simulink model "Mpc_SimMechanics_with_standing"  (R2017b)
settings: Solver=ode45  StartTime=0  StopTime=10  FixedStep=0.0005  EnableMultiTasking=on
InitFcn:
  | isSim = 1;
  | 
  | PreFunctions.CustomInitFcn_with_standing;
  | PreFunctions.simulationInitFcn_with_standing;
undefined symbols (not defined in the file): alpha_x, alpha_y, DiagnosticCodes, DynamicMatrixLibrary, motorPositions, motorVelocities, pelvisPosition, pelvisVelocity, sample_time, X, Y, Z
libraries: sm_lib x170, nesl_utility x75, Contact_Forces_Lib x6, ComponentLibrary x5, xpcrtudplib x2, slrtlib x1
(part 8 of 8)

== system Mpc_SimMechanics_with_standing/Cassie/Cassie Simulation/Cassie Right Leg/Hip Roll Drive ==
  Bus Element In : Inport  PortName=InBus  Element=torque
  Actual Torque Scaling : Gain  Gain=-gearRatio
  Constant1 : Constant  Value=0
  Constant2 : Constant  Value=0  OutDataTypeStr=uint16
  Constant3 : Constant  Value=0
  Constant4 : Constant  Value=peakTorque*gearRatio
  Constant5 : Constant  Value=gearRatio
  Gear Constraint : sm_lib/Gears and Couplings/Gears/Common Gear Constraint  GearType=External  SpecificationType=CenterDistanceRatio  CenterDistance=1e-6  CenterDistanceUnits=m  GearRatio=gearRatio  BaseGearRadius=10.0  BaseGearRadiusUnits=cm  FollGearRadius=10.0  FollGearRadiusUnits=cm  AssemblyGearRotation=Free
      settings: SourceProductName=Simscape Multibody  SourceProductBaseCode=MS
  Gear Constraint Offset : sm_lib/Frames and Transforms/Rigid Transform  TranslationMethod=StandardAxis  TranslationStandardOffset=1e-6  TranslationLengthUnit=m  TranslationStandardAxis=+Y  TranslationCartesianOffset=[0 0 0]  TranslationROffset=0  TranslationROffsetUnits=m  TranslationZOffset=0  TranslationZOffsetUnits=m  TranslationThetaOffset=0  TranslationThetaOffsetUnits=deg  RotationMethod=None  RotationAngleUnits=deg  RotationStandardAxis=+Z  RotationAngle=0.0  RotationArbitraryAxis=[0 0 1]  FollAlignAxisA=+X  BaseAlignAxisA=+Y  FollAlignAxisB=+Y  BaseAlignAxisB=+Z  RotationSequenceAxes=FollowerAxes  RotationSequence=XYX  RotationSequenceAngles=[0 0 0]  RotationSequenceAnglesUnits=deg  RotationMatrix=[1 0 0; 0 1 0; 0 0 1]
  Input Revolute Joint : sm_lib/Joints/Revolute Joint  SenseConstraintForce=off  SenseConstraintForceX=off  SenseConstraintForceY=off  SenseConstraintForceZ=off  SenseConstraintTorque=off  SenseConstraintTorqueX=off  SenseConstraintTorqueY=off  SenseConstraintTorqueZ=off  SenseTotalForce=off  SenseTotalForceX=off  SenseTotalForceY=off  SenseTotalForceZ=off  SenseTotalTorque=off  SenseTotalTorqueX=off  SenseTotalTorqueY=off  SenseTotalTorqueZ=off  CompositeWrenchDir=FollowerOnBase  CompositeWrenchFrame=BaseFrame  EquilibriumPosition=0  EquilibriumPositionUnits=rad  SpringStiffness=0  SpringStiffnessUnits=N*m/rad  DampingCoefficient=0  DampingCoefficientUnits=N*m/(rad/s)  TorqueActuationMode=InputTorque  MotionActuationMode=ComputedMotion  SensePosition=off  SenseVelocity=on  SenseAcceleration=off  SenseTorqueForce=off  PositionTargetSpecify=off  PositionTargetPriority=High  PositionTargetValue=0  PositionTargetValueUnits=deg  VelocityTargetSpecify=off  VelocityTargetPriority=High  VelocityTargetValue=0  VelocityTargetValueUnits=rad/s
  MATLAB Function : MATLAB Function  TreatAsAtomicUnit=on
  Output Revolute Joint : sm_lib/Joints/Revolute Joint  SenseConstraintForce=off  SenseConstraintForceX=off  SenseConstraintForceY=off  SenseConstraintForceZ=off  SenseConstraintTorque=off  SenseConstraintTorqueX=off  SenseConstraintTorqueY=off  SenseConstraintTorqueZ=off  SenseTotalForce=off  SenseTotalForceX=off  SenseTotalForceY=off  SenseTotalForceZ=off  SenseTotalTorque=off  SenseTotalTorqueX=off  SenseTotalTorqueY=off  SenseTotalTorqueZ=off  CompositeWrenchDir=FollowerOnBase  CompositeWrenchFrame=BaseFrame  EquilibriumPosition=0  EquilibriumPositionUnits=rad  SpringStiffness=0  SpringStiffnessUnits=N*m/rad  DampingCoefficient=1  DampingCoefficientUnits=N*m/(rad/s)  TorqueActuationMode=NoTorque  MotionActuationMode=ComputedMotion  SensePosition=on  SenseVelocity=on  SenseAcceleration=off  SenseTorqueForce=off  PositionTargetSpecify=on  PositionTargetPriority=High  PositionTargetValue=initialPosition  PositionTargetValueUnits=rad  VelocityTargetSpecify=on  VelocityTargetPriority=High  VelocityTargetValue=initialVelocity  VelocityTargetValueUnits=rad/s
  PS-Simulink Converter : nesl_utility/PS-Simulink Converter  PhysicalDomain=network_engine_domain  SubClassName=ps_output  LeftPortType=input  RightPortType=output  PseudoPeriodic=off  Frequencies=[]  Unit=rad  AffineConversion=off
  PS-Simulink Converter1 : nesl_utility/PS-Simulink Converter  PhysicalDomain=network_engine_domain  SubClassName=ps_output  LeftPortType=input  RightPortType=output  PseudoPeriodic=off  Frequencies=[]  Unit=rad/s  AffineConversion=off
  PS-Simulink Converter2 : nesl_utility/PS-Simulink Converter  PhysicalDomain=network_engine_domain  SubClassName=ps_output  LeftPortType=input  RightPortType=output  PseudoPeriodic=off  Frequencies=[]  Unit=rad/s  AffineConversion=off
  Quantizer : Quantizer  QuantizationInterval=(2*pi)/(encoderResolution*gearRatio)
  Rate Transition : RateTransition  Deterministic=off  InitialCondition=initialPosition  OutPortSampleTimeOpt=Inherit
  Rate Transition1 : RateTransition  Deterministic=off  InitialCondition=initialPosition  OutPortSampleTimeOpt=Inherit
  Rotor Solid : sm_lib/Body Elements/Solid  InertiaType=Custom  Mass=0  MassUnits=kg  CenterOfMass=[0; 0; 0]  CenterOfMassUnits=m  MomentsOfInertia=[0; 0; rotorInertia]  MomentsOfInertiaUnits=kg*m^2  ProductsOfInertia=[0; 0; 0]  ProductsOfInertiaUnits=kg*m^2  DensityBased=on  Density=1000  DensityUnits=kg/m^3  DoExposeReferenceFrame=on  SerializedFrames=<Frames/>  GraphicType=None  MarkerShape=Sphere  MarkerSize=10  GraphicVisPropType=SimpleVisualProperties  GraphicDiffuseColor=[0.5 0.5 0.5]  GraphicSpecularColor=[0.5 0.5 0.5 1.0]  GraphicAmbientColor=[0.15 0.15 0.15 1.0]  GraphicEmissiveColor=[0.0 0.0 0.0 1.0]  GraphicShininess=75  GraphicOpacity=1.0  GeometryShape=Cylinder  RectangleSize=[1 1]  RectangleSizeUnits=m  BrickDimensions=[1 1 1]  BrickDimensionUnits=m  CylinderRadius=1  CylinderRadiusUnits=m  CylinderLength=1  CylinderLengthUnits=m  SphereRadius=1  SphereRadiusUnits=m  EllipsoidRadii=[1 1 1]  EllipsoidRadiiUnits=m  ExtrusionCrossSection=[1 1; -1 1; -1 -1; 1 -1]  ExtrusionCrossSectionUnits=m  ExtrusionLength=1  ExtrusionLengthUnits=m  PolygonNumSides=3  PolygonOuterRadius=1  PolygonOuterRadiusUnits=m  ExtGeomFileType=STEP  ExtGeomFileUnits=m  RevolutionCrossSection=[1 1; 1 -1; 2 -1; 2 1]  RevolutionCrossSectionUnits=m  RevolutionExtent=Full  RevolutionAngle=180  RevolutionAngleUnits=deg
  Simulink-PS Converter : nesl_utility/Simulink-PS Converter  PhysicalDomain=network_engine_domain  SubClassName=ps_input  LeftPortType=input  RightPortType=output  PseudoPeriodic=off  Frequencies=[]  NoiseDistribution=none  NoiseParameters=[]  Unit=N*m  AffineConversion=off  FilteringAndDerivatives=zero  SimscapeFilterOrder=1  InputFilterTimeConstant=0.001  UdotUserProvided=1
  Target Torque Scaling : Gain  Gain=-1/gearRatio
  Base : PMIOPort  Port=1  Side=Left
  Follower : PMIOPort  Port=2  Side=Right
  Bus Element Out3 : Outport  PortName=OutBus  Element=statusWord
  Bus Element Out : Outport  PortName=OutBus  Element=position
  Bus Element Out4 : Outport  PortName=OutBus  Element=velocity
  Bus Element Out2 : Outport  PortName=OutBus  Element=torque
  Bus Element Out1 : Outport  PortName=OutBus  Element=driveTemperature
  Bus Element Out5 : Outport  PortName=OutBus  Element=dcLinkVoltage
  Bus Element Out6 : Outport  PortName=OutBus  Element=torqueLimit
  Bus Element Out7 : Outport  PortName=OutBus  Element=gearRatio
  Pos : Outport  Port=2
  vel : Outport  Port=3
  wires:
  PS-Simulink Converter2/1 -> vel/1, Rate Transition1/1
  Rate Transition1/1 -> Bus Element Out4/1
  Constant5/1 -> Bus Element Out7/1
  Actual Torque Scaling/1 -> Bus Element Out2/1
  Constant4/1 -> Bus Element Out6/1
  Constant3/1 -> Bus Element Out5/1
  Constant1/1 -> Bus Element Out1/1
  Constant2/1 -> Bus Element Out3/1
  Target Torque Scaling/1 -> MATLAB Function/2("torque ")
  PS-Simulink Converter1/1 -> MATLAB Function/1(speed)
  MATLAB Function/1(torque) -> Simulink-PS Converter/1, Actual Torque Scaling/1
  Bus Element In/1 -> Target Torque Scaling/1
  Quantizer/1 -> Bus Element Out/1
  PS-Simulink Converter/1 -> Pos/1, Rate Transition/1
  Rate Transition/1 -> Quantizer/1
  connections:
  Output Revolute Joint/RConn3 -- PS-Simulink Converter2/LConn1
  Input Revolute Joint/LConn1 -- Base/RConn1 -- Gear Constraint Offset/LConn1
  Simulink-PS Converter/RConn1 -- Input Revolute Joint/LConn2
  PS-Simulink Converter1/LConn1 -- Input Revolute Joint/RConn2
  Rotor Solid/RConn1 -- Gear Constraint/LConn1 -- Input Revolute Joint/RConn1
  Output Revolute Joint/RConn1 -- Follower/RConn1 -- Gear Constraint/RConn1
  Output Revolute Joint/LConn1 -- Gear Constraint Offset/RConn1
  Output Revolute Joint/RConn2 -- PS-Simulink Converter/LConn1

== system Mpc_SimMechanics_with_standing/Cassie/Cassie Simulation/Cassie Right Leg/Hip Yaw Drive ==
  Bus Element In : Inport  PortName=InBus  Element=torque
  Actual Torque Scaling : Gain  Gain=-gearRatio
  Constant1 : Constant  Value=0
  Constant2 : Constant  Value=0  OutDataTypeStr=uint16
  Constant3 : Constant  Value=0
  Constant4 : Constant  Value=peakTorque*gearRatio
  Constant5 : Constant  Value=gearRatio
  Gear Constraint : sm_lib/Gears and Couplings/Gears/Common Gear Constraint  GearType=External  SpecificationType=CenterDistanceRatio  CenterDistance=1e-6  CenterDistanceUnits=m  GearRatio=gearRatio  BaseGearRadius=10.0  BaseGearRadiusUnits=cm  FollGearRadius=10.0  FollGearRadiusUnits=cm  AssemblyGearRotation=Free
      settings: SourceProductName=Simscape Multibody  SourceProductBaseCode=MS
  Gear Constraint Offset : sm_lib/Frames and Transforms/Rigid Transform  TranslationMethod=StandardAxis  TranslationStandardOffset=1e-6  TranslationLengthUnit=m  TranslationStandardAxis=+Y  TranslationCartesianOffset=[0 0 0]  TranslationROffset=0  TranslationROffsetUnits=m  TranslationZOffset=0  TranslationZOffsetUnits=m  TranslationThetaOffset=0  TranslationThetaOffsetUnits=deg  RotationMethod=None  RotationAngleUnits=deg  RotationStandardAxis=+Z  RotationAngle=0.0  RotationArbitraryAxis=[0 0 1]  FollAlignAxisA=+X  BaseAlignAxisA=+Y  FollAlignAxisB=+Y  BaseAlignAxisB=+Z  RotationSequenceAxes=FollowerAxes  RotationSequence=XYX  RotationSequenceAngles=[0 0 0]  RotationSequenceAnglesUnits=deg  RotationMatrix=[1 0 0; 0 1 0; 0 0 1]
  Input Revolute Joint : sm_lib/Joints/Revolute Joint  SenseConstraintForce=off  SenseConstraintForceX=off  SenseConstraintForceY=off  SenseConstraintForceZ=off  SenseConstraintTorque=off  SenseConstraintTorqueX=off  SenseConstraintTorqueY=off  SenseConstraintTorqueZ=off  SenseTotalForce=off  SenseTotalForceX=off  SenseTotalForceY=off  SenseTotalForceZ=off  SenseTotalTorque=off  SenseTotalTorqueX=off  SenseTotalTorqueY=off  SenseTotalTorqueZ=off  CompositeWrenchDir=FollowerOnBase  CompositeWrenchFrame=BaseFrame  EquilibriumPosition=0  EquilibriumPositionUnits=rad  SpringStiffness=0  SpringStiffnessUnits=N*m/rad  DampingCoefficient=0  DampingCoefficientUnits=N*m/(rad/s)  TorqueActuationMode=InputTorque  MotionActuationMode=ComputedMotion  SensePosition=off  SenseVelocity=on  SenseAcceleration=off  SenseTorqueForce=off  PositionTargetSpecify=off  PositionTargetPriority=High  PositionTargetValue=0  PositionTargetValueUnits=deg  VelocityTargetSpecify=off  VelocityTargetPriority=High  VelocityTargetValue=0  VelocityTargetValueUnits=rad/s
  MATLAB Function : MATLAB Function  TreatAsAtomicUnit=on
  Output Revolute Joint : sm_lib/Joints/Revolute Joint  SenseConstraintForce=off  SenseConstraintForceX=off  SenseConstraintForceY=off  SenseConstraintForceZ=off  SenseConstraintTorque=off  SenseConstraintTorqueX=off  SenseConstraintTorqueY=off  SenseConstraintTorqueZ=off  SenseTotalForce=off  SenseTotalForceX=off  SenseTotalForceY=off  SenseTotalForceZ=off  SenseTotalTorque=off  SenseTotalTorqueX=off  SenseTotalTorqueY=off  SenseTotalTorqueZ=off  CompositeWrenchDir=FollowerOnBase  CompositeWrenchFrame=BaseFrame  EquilibriumPosition=0  EquilibriumPositionUnits=rad  SpringStiffness=0  SpringStiffnessUnits=N*m/rad  DampingCoefficient=1  DampingCoefficientUnits=N*m/(rad/s)  TorqueActuationMode=NoTorque  MotionActuationMode=ComputedMotion  SensePosition=on  SenseVelocity=on  SenseAcceleration=off  SenseTorqueForce=off  PositionTargetSpecify=on  PositionTargetPriority=High  PositionTargetValue=initialPosition  PositionTargetValueUnits=rad  VelocityTargetSpecify=on  VelocityTargetPriority=High  VelocityTargetValue=initialVelocity  VelocityTargetValueUnits=rad/s
  PS-Simulink Converter : nesl_utility/PS-Simulink Converter  PhysicalDomain=network_engine_domain  SubClassName=ps_output  LeftPortType=input  RightPortType=output  PseudoPeriodic=off  Frequencies=[]  Unit=rad  AffineConversion=off
  PS-Simulink Converter1 : nesl_utility/PS-Simulink Converter  PhysicalDomain=network_engine_domain  SubClassName=ps_output  LeftPortType=input  RightPortType=output  PseudoPeriodic=off  Frequencies=[]  Unit=rad/s  AffineConversion=off
  PS-Simulink Converter2 : nesl_utility/PS-Simulink Converter  PhysicalDomain=network_engine_domain  SubClassName=ps_output  LeftPortType=input  RightPortType=output  PseudoPeriodic=off  Frequencies=[]  Unit=rad/s  AffineConversion=off
  Quantizer : Quantizer  QuantizationInterval=(2*pi)/(encoderResolution*gearRatio)
  Rate Transition : RateTransition  Deterministic=off  InitialCondition=initialPosition  OutPortSampleTimeOpt=Inherit
  Rate Transition1 : RateTransition  Deterministic=off  InitialCondition=initialPosition  OutPortSampleTimeOpt=Inherit
  Rotor Solid : sm_lib/Body Elements/Solid  InertiaType=Custom  Mass=0  MassUnits=kg  CenterOfMass=[0; 0; 0]  CenterOfMassUnits=m  MomentsOfInertia=[0; 0; rotorInertia]  MomentsOfInertiaUnits=kg*m^2  ProductsOfInertia=[0; 0; 0]  ProductsOfInertiaUnits=kg*m^2  DensityBased=on  Density=1000  DensityUnits=kg/m^3  DoExposeReferenceFrame=on  SerializedFrames=<Frames/>  GraphicType=None  MarkerShape=Sphere  MarkerSize=10  GraphicVisPropType=SimpleVisualProperties  GraphicDiffuseColor=[0.5 0.5 0.5]  GraphicSpecularColor=[0.5 0.5 0.5 1.0]  GraphicAmbientColor=[0.15 0.15 0.15 1.0]  GraphicEmissiveColor=[0.0 0.0 0.0 1.0]  GraphicShininess=75  GraphicOpacity=1.0  GeometryShape=Cylinder  RectangleSize=[1 1]  RectangleSizeUnits=m  BrickDimensions=[1 1 1]  BrickDimensionUnits=m  CylinderRadius=1  CylinderRadiusUnits=m  CylinderLength=1  CylinderLengthUnits=m  SphereRadius=1  SphereRadiusUnits=m  EllipsoidRadii=[1 1 1]  EllipsoidRadiiUnits=m  ExtrusionCrossSection=[1 1; -1 1; -1 -1; 1 -1]  ExtrusionCrossSectionUnits=m  ExtrusionLength=1  ExtrusionLengthUnits=m  PolygonNumSides=3  PolygonOuterRadius=1  PolygonOuterRadiusUnits=m  ExtGeomFileType=STEP  ExtGeomFileUnits=m  RevolutionCrossSection=[1 1; 1 -1; 2 -1; 2 1]  RevolutionCrossSectionUnits=m  RevolutionExtent=Full  RevolutionAngle=180  RevolutionAngleUnits=deg
  Simulink-PS Converter : nesl_utility/Simulink-PS Converter  PhysicalDomain=network_engine_domain  SubClassName=ps_input  LeftPortType=input  RightPortType=output  PseudoPeriodic=off  Frequencies=[]  NoiseDistribution=none  NoiseParameters=[]  Unit=N*m  AffineConversion=off  FilteringAndDerivatives=zero  SimscapeFilterOrder=1  InputFilterTimeConstant=0.001  UdotUserProvided=1
  Target Torque Scaling : Gain  Gain=-1/gearRatio
  Base : PMIOPort  Port=1  Side=Left
  Follower : PMIOPort  Port=2  Side=Right
  Bus Element Out3 : Outport  PortName=OutBus  Element=statusWord
  Bus Element Out : Outport  PortName=OutBus  Element=position
  Bus Element Out4 : Outport  PortName=OutBus  Element=velocity
  Bus Element Out2 : Outport  PortName=OutBus  Element=torque
  Bus Element Out1 : Outport  PortName=OutBus  Element=driveTemperature
  Bus Element Out5 : Outport  PortName=OutBus  Element=dcLinkVoltage
  Bus Element Out6 : Outport  PortName=OutBus  Element=torqueLimit
  Bus Element Out7 : Outport  PortName=OutBus  Element=gearRatio
  Pos : Outport  Port=2
  vel : Outport  Port=3
  wires:
  PS-Simulink Converter2/1 -> vel/1, Rate Transition1/1
  Rate Transition1/1 -> Bus Element Out4/1
  Constant5/1 -> Bus Element Out7/1
  Actual Torque Scaling/1 -> Bus Element Out2/1
  Constant4/1 -> Bus Element Out6/1
  Constant3/1 -> Bus Element Out5/1
  Constant1/1 -> Bus Element Out1/1
  Constant2/1 -> Bus Element Out3/1
  Target Torque Scaling/1 -> MATLAB Function/2("torque ")
  PS-Simulink Converter1/1 -> MATLAB Function/1(speed)
  MATLAB Function/1(torque) -> Simulink-PS Converter/1, Actual Torque Scaling/1
  Bus Element In/1 -> Target Torque Scaling/1
  Quantizer/1 -> Bus Element Out/1
  PS-Simulink Converter/1 -> Pos/1, Rate Transition/1
  Rate Transition/1 -> Quantizer/1
  connections:
  Output Revolute Joint/RConn3 -- PS-Simulink Converter2/LConn1
  Input Revolute Joint/LConn1 -- Base/RConn1 -- Gear Constraint Offset/LConn1
  Simulink-PS Converter/RConn1 -- Input Revolute Joint/LConn2
  PS-Simulink Converter1/LConn1 -- Input Revolute Joint/RConn2
  Rotor Solid/RConn1 -- Gear Constraint/LConn1 -- Input Revolute Joint/RConn1
  Output Revolute Joint/RConn1 -- Follower/RConn1 -- Gear Constraint/RConn1
  Output Revolute Joint/LConn1 -- Gear Constraint Offset/RConn1
  Output Revolute Joint/RConn2 -- PS-Simulink Converter/LConn1

== system Mpc_SimMechanics_with_standing/Cassie/Cassie Simulation/Cassie Right Leg/Knee Drive ==
  Bus Element In : Inport  PortName=InBus  Element=torque
  Actual Torque Scaling : Gain  Gain=-gearRatio
  Constant1 : Constant  Value=0
  Constant2 : Constant  Value=0  OutDataTypeStr=uint16
  Constant3 : Constant  Value=0
  Constant4 : Constant  Value=peakTorque*gearRatio
  Constant5 : Constant  Value=gearRatio
  Gear Constraint : sm_lib/Gears and Couplings/Gears/Common Gear Constraint  GearType=External  SpecificationType=CenterDistanceRatio  CenterDistance=1e-6  CenterDistanceUnits=m  GearRatio=gearRatio  BaseGearRadius=10.0  BaseGearRadiusUnits=cm  FollGearRadius=10.0  FollGearRadiusUnits=cm  AssemblyGearRotation=Free
      settings: SourceProductName=Simscape Multibody  SourceProductBaseCode=MS
  Gear Constraint Offset : sm_lib/Frames and Transforms/Rigid Transform  TranslationMethod=StandardAxis  TranslationStandardOffset=1e-6  TranslationLengthUnit=m  TranslationStandardAxis=+Y  TranslationCartesianOffset=[0 0 0]  TranslationROffset=0  TranslationROffsetUnits=m  TranslationZOffset=0  TranslationZOffsetUnits=m  TranslationThetaOffset=0  TranslationThetaOffsetUnits=deg  RotationMethod=None  RotationAngleUnits=deg  RotationStandardAxis=+Z  RotationAngle=0.0  RotationArbitraryAxis=[0 0 1]  FollAlignAxisA=+X  BaseAlignAxisA=+Y  FollAlignAxisB=+Y  BaseAlignAxisB=+Z  RotationSequenceAxes=FollowerAxes  RotationSequence=XYX  RotationSequenceAngles=[0 0 0]  RotationSequenceAnglesUnits=deg  RotationMatrix=[1 0 0; 0 1 0; 0 0 1]
  Input Revolute Joint : sm_lib/Joints/Revolute Joint  SenseConstraintForce=off  SenseConstraintForceX=off  SenseConstraintForceY=off  SenseConstraintForceZ=off  SenseConstraintTorque=off  SenseConstraintTorqueX=off  SenseConstraintTorqueY=off  SenseConstraintTorqueZ=off  SenseTotalForce=off  SenseTotalForceX=off  SenseTotalForceY=off  SenseTotalForceZ=off  SenseTotalTorque=off  SenseTotalTorqueX=off  SenseTotalTorqueY=off  SenseTotalTorqueZ=off  CompositeWrenchDir=FollowerOnBase  CompositeWrenchFrame=BaseFrame  EquilibriumPosition=0  EquilibriumPositionUnits=rad  SpringStiffness=0  SpringStiffnessUnits=N*m/rad  DampingCoefficient=0  DampingCoefficientUnits=N*m/(rad/s)  TorqueActuationMode=InputTorque  MotionActuationMode=ComputedMotion  SensePosition=off  SenseVelocity=on  SenseAcceleration=off  SenseTorqueForce=off  PositionTargetSpecify=off  PositionTargetPriority=High  PositionTargetValue=0  PositionTargetValueUnits=deg  VelocityTargetSpecify=off  VelocityTargetPriority=High  VelocityTargetValue=0  VelocityTargetValueUnits=rad/s
  MATLAB Function : MATLAB Function  TreatAsAtomicUnit=on
  Output Revolute Joint : sm_lib/Joints/Revolute Joint  SenseConstraintForce=off  SenseConstraintForceX=off  SenseConstraintForceY=off  SenseConstraintForceZ=off  SenseConstraintTorque=off  SenseConstraintTorqueX=off  SenseConstraintTorqueY=off  SenseConstraintTorqueZ=off  SenseTotalForce=off  SenseTotalForceX=off  SenseTotalForceY=off  SenseTotalForceZ=off  SenseTotalTorque=off  SenseTotalTorqueX=off  SenseTotalTorqueY=off  SenseTotalTorqueZ=off  CompositeWrenchDir=FollowerOnBase  CompositeWrenchFrame=BaseFrame  EquilibriumPosition=0  EquilibriumPositionUnits=rad  SpringStiffness=0  SpringStiffnessUnits=N*m/rad  DampingCoefficient=1  DampingCoefficientUnits=N*m/(rad/s)  TorqueActuationMode=NoTorque  MotionActuationMode=ComputedMotion  SensePosition=on  SenseVelocity=on  SenseAcceleration=off  SenseTorqueForce=off  PositionTargetSpecify=on  PositionTargetPriority=High  PositionTargetValue=initialPosition  PositionTargetValueUnits=rad  VelocityTargetSpecify=on  VelocityTargetPriority=High  VelocityTargetValue=initialVelocity  VelocityTargetValueUnits=rad/s
  PS-Simulink Converter : nesl_utility/PS-Simulink Converter  PhysicalDomain=network_engine_domain  SubClassName=ps_output  LeftPortType=input  RightPortType=output  PseudoPeriodic=off  Frequencies=[]  Unit=rad  AffineConversion=off
  PS-Simulink Converter1 : nesl_utility/PS-Simulink Converter  PhysicalDomain=network_engine_domain  SubClassName=ps_output  LeftPortType=input  RightPortType=output  PseudoPeriodic=off  Frequencies=[]  Unit=rad/s  AffineConversion=off
  PS-Simulink Converter2 : nesl_utility/PS-Simulink Converter  PhysicalDomain=network_engine_domain  SubClassName=ps_output  LeftPortType=input  RightPortType=output  PseudoPeriodic=off  Frequencies=[]  Unit=rad/s  AffineConversion=off
  Quantizer : Quantizer  QuantizationInterval=(2*pi)/(encoderResolution*gearRatio)
  Rate Transition : RateTransition  Deterministic=off  InitialCondition=initialPosition  OutPortSampleTimeOpt=Inherit
  Rate Transition1 : RateTransition  Deterministic=off  InitialCondition=initialPosition  OutPortSampleTimeOpt=Inherit
  Rotor Solid : sm_lib/Body Elements/Solid  InertiaType=Custom  Mass=0  MassUnits=kg  CenterOfMass=[0; 0; 0]  CenterOfMassUnits=m  MomentsOfInertia=[0; 0; rotorInertia]  MomentsOfInertiaUnits=kg*m^2  ProductsOfInertia=[0; 0; 0]  ProductsOfInertiaUnits=kg*m^2  DensityBased=on  Density=1000  DensityUnits=kg/m^3  DoExposeReferenceFrame=on  SerializedFrames=<Frames/>  GraphicType=None  MarkerShape=Sphere  MarkerSize=10  GraphicVisPropType=SimpleVisualProperties  GraphicDiffuseColor=[0.5 0.5 0.5]  GraphicSpecularColor=[0.5 0.5 0.5 1.0]  GraphicAmbientColor=[0.15 0.15 0.15 1.0]  GraphicEmissiveColor=[0.0 0.0 0.0 1.0]  GraphicShininess=75  GraphicOpacity=1.0  GeometryShape=Cylinder  RectangleSize=[1 1]  RectangleSizeUnits=m  BrickDimensions=[1 1 1]  BrickDimensionUnits=m  CylinderRadius=1  CylinderRadiusUnits=m  CylinderLength=1  CylinderLengthUnits=m  SphereRadius=1  SphereRadiusUnits=m  EllipsoidRadii=[1 1 1]  EllipsoidRadiiUnits=m  ExtrusionCrossSection=[1 1; -1 1; -1 -1; 1 -1]  ExtrusionCrossSectionUnits=m  ExtrusionLength=1  ExtrusionLengthUnits=m  PolygonNumSides=3  PolygonOuterRadius=1  PolygonOuterRadiusUnits=m  ExtGeomFileType=STEP  ExtGeomFileUnits=m  RevolutionCrossSection=[1 1; 1 -1; 2 -1; 2 1]  RevolutionCrossSectionUnits=m  RevolutionExtent=Full  RevolutionAngle=180  RevolutionAngleUnits=deg
  Simulink-PS Converter : nesl_utility/Simulink-PS Converter  PhysicalDomain=network_engine_domain  SubClassName=ps_input  LeftPortType=input  RightPortType=output  PseudoPeriodic=off  Frequencies=[]  NoiseDistribution=none  NoiseParameters=[]  Unit=N*m  AffineConversion=off  FilteringAndDerivatives=zero  SimscapeFilterOrder=1  InputFilterTimeConstant=0.001  UdotUserProvided=1
  Target Torque Scaling : Gain  Gain=-1/gearRatio
  Base : PMIOPort  Port=1  Side=Left
  Follower : PMIOPort  Port=2  Side=Right
  Bus Element Out3 : Outport  PortName=OutBus  Element=statusWord
  Bus Element Out : Outport  PortName=OutBus  Element=position
  Bus Element Out4 : Outport  PortName=OutBus  Element=velocity
  Bus Element Out2 : Outport  PortName=OutBus  Element=torque
  Bus Element Out1 : Outport  PortName=OutBus  Element=driveTemperature
  Bus Element Out5 : Outport  PortName=OutBus  Element=dcLinkVoltage
  Bus Element Out6 : Outport  PortName=OutBus  Element=torqueLimit
  Bus Element Out7 : Outport  PortName=OutBus  Element=gearRatio
  Pos : Outport  Port=2
  vel : Outport  Port=3
  wires:
  PS-Simulink Converter2/1 -> vel/1, Rate Transition1/1
  Rate Transition1/1 -> Bus Element Out4/1
  Constant5/1 -> Bus Element Out7/1
  Actual Torque Scaling/1 -> Bus Element Out2/1
  Constant4/1 -> Bus Element Out6/1
  Constant3/1 -> Bus Element Out5/1
  Constant1/1 -> Bus Element Out1/1
  Constant2/1 -> Bus Element Out3/1
  Target Torque Scaling/1 -> MATLAB Function/2("torque ")
  PS-Simulink Converter1/1 -> MATLAB Function/1(speed)
  MATLAB Function/1(torque) -> Simulink-PS Converter/1, Actual Torque Scaling/1
  Bus Element In/1 -> Target Torque Scaling/1
  Quantizer/1 -> Bus Element Out/1
  PS-Simulink Converter/1 -> Pos/1, Rate Transition/1
  Rate Transition/1 -> Quantizer/1
  connections:
  Output Revolute Joint/RConn3 -- PS-Simulink Converter2/LConn1
  Input Revolute Joint/LConn1 -- Base/RConn1 -- Gear Constraint Offset/LConn1
  Simulink-PS Converter/RConn1 -- Input Revolute Joint/LConn2
  PS-Simulink Converter1/LConn1 -- Input Revolute Joint/RConn2
  Rotor Solid/RConn1 -- Gear Constraint/LConn1 -- Input Revolute Joint/RConn1
  Output Revolute Joint/RConn1 -- Follower/RConn1 -- Gear Constraint/RConn1
  Output Revolute Joint/LConn1 -- Gear Constraint Offset/RConn1
  Output Revolute Joint/RConn2 -- PS-Simulink Converter/LConn1

== matlab function Mpc_SimMechanics_with_standing/Cassie/Cassie Simulation/World/MATLAB Function ==
  data: px input; vx input; fx output; py input; vy input; pz input; vz input; fy output; fz output; t input
function [fx,fy,fz] = fcn(px,vx,py,vy,pz,vz,t)
P = 100000;
D = 1000;
fx = 0; fy = 0; fz = 0;
% if t<0.1
% fx = -P*px - D*vx;
% fy = -P*py - D*vy;
% fz = - 10000*vz;
% end

% if t > 6 && t <6.2
% fx = -20;
% end

== matlab function Mpc_SimMechanics_with_standing/Cassie/Cassie Simulation/Cassie Left Leg/Knee Drive/MATLAB Function ==
  data: speed input; torque output; torque input; peakTorque parameter; peakSpeed parameter
function torque = fcn(speed, torque, peakTorque, peakSpeed) %#codegen

  % Cap the velocity at the specified limits to avoid extrapolation
  speed = median([-peakSpeed, speed, peakSpeed]);

  % Linear interpolation of speed-torque curve
  torqueLimit = interp1(...
    [0, 0.5*peakSpeed, peakSpeed], ...
    [peakTorque, peakTorque, 0], ...
    abs(speed));

  % Cap the torque command at the specified imits
  torque = median([-torqueLimit, torque, torqueLimit]);
end % fcn

== matlab function Mpc_SimMechanics_with_standing/Cassie/Cassie Simulation/Cassie Pelvis/VectorNav/World Acceleration to Accelerometer Measurement1 ==
  data: q input; a1 output; a input
function a1 = fcn(q, a)
  % Construct quaternion object
  Q = Quaternion(q);
  
  % Add world gravity acceleration to body acceleration
  a1 = Q.getRotation.getValue'*(a + [0; 0; -9.806]);
end % fcn

== matlab function Mpc_SimMechanics_with_standing/Cassie/Cassie Simulation/Cassie Left Leg/Hip Roll Drive/MATLAB Function ==
  data: speed input; torque output; torque input; peakTorque parameter; peakSpeed parameter
function torque = fcn(speed, torque, peakTorque, peakSpeed) %#codegen

  % Cap the velocity at the specified limits to avoid extrapolation
  speed = median([-peakSpeed, speed, peakSpeed]);

  % Linear interpolation of speed-torque curve
  torqueLimit = interp1(...
    [0, 0.5*peakSpeed, peakSpeed], ...
    [peakTorque, peakTorque, 0], ...
    abs(speed));

  % Cap the torque command at the specified imits
  torque = median([-torqueLimit, torque, torqueLimit]);
end % fcn

== matlab function Mpc_SimMechanics_with_standing/Cassie/Cassie Simulation/Cassie Left Leg/Hip Yaw Drive/MATLAB Function ==
  data: speed input; torque output; torque input; peakTorque parameter; peakSpeed parameter
function torque = fcn(speed, torque, peakTorque, peakSpeed) %#codegen

  % Cap the velocity at the specified limits to avoid extrapolation
  speed = median([-peakSpeed, speed, peakSpeed]);

  % Linear interpolation of speed-torque curve
  torqueLimit = interp1(...
    [0, 0.5*peakSpeed, peakSpeed], ...
    [peakTorque, peakTorque, 0], ...
    abs(speed));

  % Cap the torque command at the specified imits
  torque = median([-torqueLimit, torque, torqueLimit]);
end % fcn

== matlab function Mpc_SimMechanics_with_standing/Cassie/Cassie Simulation/Cassie Left Leg/Hip Pitch Drive/MATLAB Function ==
  data: speed input; torque output; torque input; peakTorque parameter; peakSpeed parameter
function torque = fcn(speed, torque, peakTorque, peakSpeed) %#codegen

  % Cap the velocity at the specified limits to avoid extrapolation
  speed = median([-peakSpeed, speed, peakSpeed]);

  % Linear interpolation of speed-torque curve
  torqueLimit = interp1(...
    [0, 0.5*peakSpeed, peakSpeed], ...
    [peakTorque, peakTorque, 0], ...
    abs(speed));

  % Cap the torque command at the specified imits
  torque = median([-torqueLimit, torque, torqueLimit]);
end % fcn

== matlab function Mpc_SimMechanics_with_standing/Cassie/Cassie Simulation/Cassie Pelvis/VectorNav/MATLAB Function ==
  data: q input; q output; preRotationMatrix parameter; postRotationMatrix parameter
function q = fcn(q, preRotationMatrix, postRotationMatrix)
  % Construct constant rotation matrix objects
  R0 = coder.const(Rotation3d(preRotationMatrix));
  R2 = coder.const(Rotation3d(postRotationMatrix));
  
  % Convert rotation matrices into constant quaternion objects
  Q0 = coder.const(R0.getQuaternion);
  Q2 = coder.const(R2.getQuaternion);
  
  % Apply pre and post rotations
  Q1 = Q0*Quaternion(q)*Q2;
  
  % Convert quaternion object to double
  q = Q1.getValue;
end % fcn

== matlab function Mpc_SimMechanics_with_standing/Cassie/Cassie Simulation/Cassie Left Leg/Foot Drive/MATLAB Function ==
  data: speed input; torque output; torque input; peakTorque parameter; peakSpeed parameter
function torque = fcn(speed, torque, peakTorque, peakSpeed) %#codegen

  % Cap the velocity at the specified limits to avoid extrapolation
  speed = median([-peakSpeed, speed, peakSpeed]);

  % Linear interpolation of speed-torque curve
  torqueLimit = interp1(...
    [0, 0.5*peakSpeed, peakSpeed], ...
    [peakTorque, peakTorque, 0], ...
    abs(speed));

  % Cap the torque command at the specified imits
  torque = median([-torqueLimit, torque, torqueLimit]);
end % fcn

== matlab function Mpc_SimMechanics_with_standing/Cassie/Cassie Simulation/Cassie Right Leg/Hip Roll Drive/MATLAB Function ==
  data: speed input; torque output; torque input; peakTorque parameter; peakSpeed parameter
function torque = fcn(speed, torque, peakTorque, peakSpeed) %#codegen

  % Cap the velocity at the specified limits to avoid extrapolation
  speed = median([-peakSpeed, speed, peakSpeed]);

  % Linear interpolation of speed-torque curve
  torqueLimit = interp1(...
    [0, 0.5*peakSpeed, peakSpeed], ...
    [peakTorque, peakTorque, 0], ...
    abs(speed));

  % Cap the torque command at the specified imits
  torque = median([-torqueLimit, torque, torqueLimit]);
end % fcn

== matlab function Mpc_SimMechanics_with_standing/Cassie/Cassie Simulation/Cassie Pelvis/VectorNav/World Acceleration to Accelerometer Measurement ==
  data: q input; a1 output; a input
function a1 = fcn(q, a)
  % Construct quaternion object
  Q = Quaternion(q);
  
  % Add world gravity acceleration to body acceleration
  a1 = Q.getRotation.getValue'*(a + [0; 0; -9.806]);
end % fcn

== matlab function Mpc_SimMechanics_with_standing/Cassie/Cassie Simulation/Cassie Right Leg/Hip Yaw Drive/MATLAB Function ==
  data: speed input; torque output; torque input; peakTorque parameter; peakSpeed parameter
function torque = fcn(speed, torque, peakTorque, peakSpeed) %#codegen

  % Cap the velocity at the specified limits to avoid extrapolation
  speed = median([-peakSpeed, speed, peakSpeed]);

  % Linear interpolation of speed-torque curve
  torqueLimit = interp1(...
    [0, 0.5*peakSpeed, peakSpeed], ...
    [peakTorque, peakTorque, 0], ...
    abs(speed));

  % Cap the torque command at the specified imits
  torque = median([-torqueLimit, torque, torqueLimit]);
end % fcn

== matlab function Mpc_SimMechanics_with_standing/Cassie/Cassie Simulation/Cassie Right Leg/Hip Pitch Drive/MATLAB Function ==
  data: speed input; torque output; torque input; peakTorque parameter; peakSpeed parameter
function torque = fcn(speed, torque, peakTorque, peakSpeed) %#codegen

  % Cap the velocity at the specified limits to avoid extrapolation
  speed = median([-peakSpeed, speed, peakSpeed]);

  % Linear interpolation of speed-torque curve
  torqueLimit = interp1(...
    [0, 0.5*peakSpeed, peakSpeed], ...
    [peakTorque, peakTorque, 0], ...
    abs(speed));

  % Cap the torque command at the specified imits
  torque = median([-torqueLimit, torque, torqueLimit]);
end % fcn

== matlab function Mpc_SimMechanics_with_standing/Cassie/Cassie Simulation/Cassie Right Leg/Knee Drive/MATLAB Function ==
  data: speed input; torque output; torque input; peakTorque parameter; peakSpeed parameter
function torque = fcn(speed, torque, peakTorque, peakSpeed) %#codegen

  % Cap the velocity at the specified limits to avoid extrapolation
  speed = median([-peakSpeed, speed, peakSpeed]);

  % Linear interpolation of speed-torque curve
  torqueLimit = interp1(...
    [0, 0.5*peakSpeed, peakSpeed], ...
    [peakTorque, peakTorque, 0], ...
    abs(speed));

  % Cap the torque command at the specified imits
  torque = median([-torqueLimit, torque, torqueLimit]);
end % fcn

== matlab function Mpc_SimMechanics_with_standing/Cassie/Cassie Simulation/Cassie Right Leg/Foot Drive/MATLAB Function ==
  data: speed input; torque output; torque input; peakTorque parameter; peakSpeed parameter
function torque = fcn(speed, torque, peakTorque, peakSpeed) %#codegen

  % Cap the velocity at the specified limits to avoid extrapolation
  speed = median([-peakSpeed, speed, peakSpeed]);

  % Linear interpolation of speed-torque curve
  torqueLimit = interp1(...
    [0, 0.5*peakSpeed, peakSpeed], ...
    [peakTorque, peakTorque, 0], ...
    abs(speed));

  % Cap the torque command at the specified imits
  torque = median([-torqueLimit, torque, torqueLimit]);
end % fcn

== matlab function Mpc_SimMechanics_with_standing/MATLAB Function ==
  data: perfect_measurement input; q_perfect output; dq_perfect output
function [q_perfect, dq_perfect] = measurement2coordinate(perfect_measurement)
LinearAccelerator = perfect_measurement(1:3);
Quaternion = perfect_measurement(4:7);
AngularVelocity = perfect_measurement(8:10);
Base_pos = perfect_measurement(11:13);
LeftLeg_pos =perfect_measurement(14:21);
RightLeg_pos =perfect_measurement(22:29);
Base_vel = perfect_measurement(30:32);
LeftLeg_vel =perfect_measurement(33:40);
RightLeg_vel =perfect_measurement(41:48);

 [qyaw, qpitch, qroll, dqyaw, dqpitch, dqroll] = IMU_to_Euler_v2(Quaternion, AngularVelocity);
 
 q_perfect = [Base_pos; qyaw;   qpitch; qroll; ...
     LeftLeg_pos(1:4); LeftLeg_pos(6:7); LeftLeg_pos(5); ...
     RightLeg_pos(1:4); RightLeg_pos(6:7); RightLeg_pos(5)];
 
dq_perfect = [Base_vel; dqyaw;   dqpitch; dqroll; ...
     LeftLeg_vel(1:4); LeftLeg_vel(6:7); LeftLeg_vel(5); ...
     RightLeg_vel(1:4); RightLeg_vel(6:7); RightLeg_vel(5)];

== matlab function Mpc_SimMechanics_with_standing/Cassie/Cassie Simulation/Cassie Pelvis/VectorNav/MATLAB Function1 ==
  data: q input; q output; preRotationMatrix parameter; postRotationMatrix parameter
function q = fcn(q, preRotationMatrix, postRotationMatrix)
  % Construct constant rotation matrix objects
  R0 = coder.const(Rotation3d(preRotationMatrix));
  R2 = coder.const(Rotation3d(postRotationMatrix));
  
  % Convert rotation matrices into constant quaternion objects
  Q0 = coder.const(R0.getQuaternion);
  Q2 = coder.const(R2.getQuaternion);
  
  % Apply pre and post rotations
  Q1 = Q0*Quaternion(q)*Q2;
  
  % Convert quaternion object to double
  q = Q1.getValue;
end % fcn

== matlab function Mpc_SimMechanics_with_standing/Controller/MATLAB Function1 ==
  data: dq input; dq output; dqxyz input; EulerRates input
function dq = mix_dq(dq,dqxyz,EulerRates)
dq(1:3) = dqxyz;
dq(4:6) = EulerRates;
